simulink model "SF007A_SysFricLrng"  (R2013b)
settings: Solver=FixedStepDiscrete  SolverMode=SingleTasking  StartTime=0.0  StopTime=1  FixedStep=0.002  RelTol=1e-3
PostLoadFcn:
  | , if any(exist('dsrtsu_mdlpostloadfcn', 'file') == [2, 3, 6]), try dsrtsu_mdlpostloadfcn('Execute', bdroot); catch fprintf('Error in PostLoadFcn (dsrtsu_mdlpostloadfcn) for model "%s":\n %s\n', bdroot, lasterr); end, end,
undefined symbols (not defined in the file): ARCHGLBPRM_100MILLISEC_SEC_F32, ARCHGLBPRM_10MILLISEC_SEC_F32, ARCHGLBPRM_180OVERPI_ULS_F32, CONV100MICROSECTOSEC_ULS_F32, FLTINJ_SYSFRICLRNG_SYSFRICOFFS, FricLrngData, HiFricNtc, HWPTNUM_CNT_U08, HWPTNUMSUB1_CNT_U08, HWVELDECDIR_ULS_U08, HWVELINCDIR_ULS_U08, IDXCALCNSCAGFAC_ULS_U08, IDXSELN1_ULS_U08, IDXSELN2_ULS_U08, IDXSELN3_ULS_U08, LRNGENASCAFAC_MILLISEC_U32, NtcSts1, SCAGFACQUARTER_CNT_F32, SCAGFACTEN_CNT_U16, SECIDXSELN_ULS_U08, SysFricLrngBasLineEolFric, SysFricLrngBasLineFric, SysFricLrngBasLineHys, SysFricLrngBasLineRngCntr, SysFricLrngEolFricDifScagFac, SysFricLrngFricChgWght, SysFricLrngFricDiagcThd, SysFricLrngFricDiagcTiThd, SysFricLrngFricHysHwAgPt, SysFricLrngGain, SysFricLrngHwPosnAuthyThd, SysFricLrngHwVelConstrLim, SysFricLrngHwVelHiLim, SysFricLrngHwVelLoLim, SysFricLrngIgnCycFricChgLim, SysFricLrngLatAHiLim, SysFricLrngLatALoLim, SysFricLrngMaskVehSpd, SysFricLrngOperMod1, SysFricLrngRngCntrThd, SysFricLrngThd, SysFricLrngTHiLim, SysFricLrngTLoLim, SysFricLrngVehSpd, SYSFRICOFFSLIM_HWNWTMTR_F32, VEHSPDPTNUM1_ULS_U08, VEHSPDPTNUM2_ULS_U08
libraries: Fil x19, simulink x17, NxtrLim x10, NxtrAbslt x3, NxtrNvM x2, FixdToFloat x2, FloatToFixd x1, LnrIntrpn x1
(part 2 of 7)

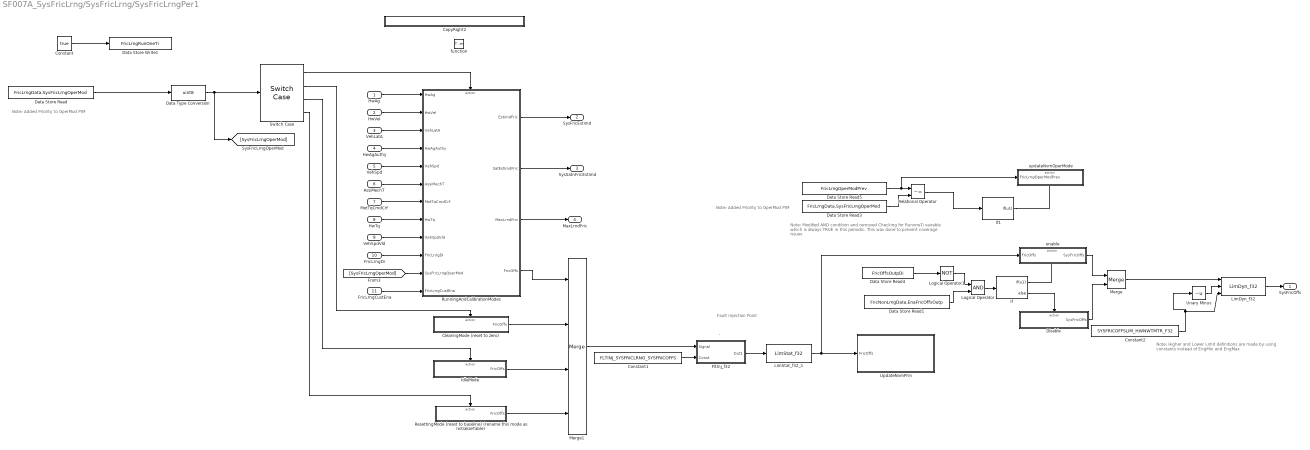
== system SF007A_SysFricLrng/SysFricLrng/SysFricLrngPer1 ==
  note: Note: Added Priority to OperMod PIM
  note: ,
  note: Fault
      | Injection
      | Point
  note: Note: Higher and Lower Limit definitions are made
      |           by using constants instead of EngMin and EngMax
  note: Note: Modified AND condition and removed Checking for RunoneTi
      | vairable which is always TRUE in this periodic. This was done to prevent
      | coverage issues
  note: Note: Added Priority to OperMod PIM
  HwAg : Inport
  HwVel : Inport  Port=2
  VehLatA : Inport  Port=3
  HwAgAuthy : Inport  Port=4
  VehSpd : Inport  Port=5
  AssiMechT : Inport  Port=6
  MotTqCmdCrf : Inport  Port=7
  HwTq : Inport  Port=8
  VehSpdVld : Inport  Port=9
  FricLrngDi : Inport  Port=10
  FricLrngCustEna : Inport  Port=11
  function : TriggerPort  TriggerType=function-call
  ClearingMode (reset to zero) : Subsystem
  Constant : Constant  Value=true  OutDataTypeStr=boolean
      settings: AttributesFormatString=%<OutDataTypeStr>
  Constant1 : Constant  Value=FLTINJ_SYSFRICLRNG_SYSFRICOFFS  SampleTime=-1
  Constant2 : Constant  Value=SYSFRICOFFSLIM_HWNWTMTR_F32  SampleTime=-1
  CopyRight2 : Subsystem  Description=|  mask(Copyright Information){none=on}
      | Copyright info block.                                               
      |                                                                     
      | Place copyright information at the top of every subsystem in design.
      mask prompts: none "No parameters"
      mask help: Place copyright information at the top of every subsystem in design.
      mask Display:
      | NxtrConf = 'Nexteer Confidential';
      | 
      | sys = bdroot; %handle for the current model ("system")
      | first = get_param(sys,'Created');
      | if(isempty(first))
      |     first = datestr(now,'yyyy');
      | else
      |     first = first(end-3:end);  %year is last four digits
      | end
      | 
      | last = get_param(sys,'LastModifiedDate');
      | if isempty(last)
      |     last = datestr(now,'yyyy');
      | else
      |     last = last(end-3:end);
      | end
      | 
      | if strcmp(first,last)
      |     fprintf('%s -- Copyright %s Nexteer',NxtrConf,first)
      | else
      |     fprintf('%s -- %s%s- %s Nexteer',NxtrConf,char(169),first,last)
      | end
  Data Store Read : DataStoreRead  Priority=1  DataStoreName=FricLrngData  DataStoreElements=FricLrngData.SysFricLrngOperMod
      settings: AttributesFormatString=Priority=%<Priority>
  Data Store Read1 : DataStoreRead  DataStoreName=FricNonLrngData  DataStoreElements=FricNonLrngData.EnaFricOffsOutp
  Data Store Read3 : DataStoreRead  Priority=2  DataStoreName=FricLrngData  DataStoreElements=FricLrngData.SysFricLrngOperMod
      settings: AttributesFormatString=Priority=%<Priority>
  Data Store Read4 : DataStoreRead  DataStoreName=FricOffsOutpDi
  Data Store Read5 : DataStoreRead  Priority=2  DataStoreName=FricLrngOperModPrev
  Data Store Write1 : DataStoreWrite  DataStoreName=FricLrngRunOneTi
  Data Type Conversion : DataTypeConversion  OutDataTypeStr=uint8
  Disable : Subsystem  TreatAsAtomicUnit=on
  FltInj_f32 : Subsystem  RequirementInfo={} %GIDa_0b9e84c1_4f47_4480_b4c5_5d0515f10b4a  TreatAsAtomicUnit=on  VariantControl=FltInj_sim  mask(Fault_Injection){}
      mask help: Fault Injection is a simulation only block for EA4 programs.
  IdleMode : Subsystem
  If : If  IfExpression=u1
  If1 : If  IfExpression=u1  ShowElse=off
  LimDyn_f32 : NxtrLim/LimDyn_f32
  LimStat_f32_1 : NxtrLim/LimStat_f32  LoLim=SysFricLrngFricOffsLoLim  HiLim=SysFricLrngFricOffsHiLim
      settings: AttributesFormatString=|
      | Low Limit: %<LoLim>
      | High Limit:%<HiLim>
  Logical Operator : Logic  AllPortsSameDT=off  OutDataTypeStr=boolean
  Logical Operator1 : Logic  Operator=NOT  AllPortsSameDT=off  OutDataTypeStr=boolean
  Merge : Merge
  Merge1 : Merge  Inputs=4
  Relational Operator : RelationalOperator  Operator=~=  OutDataTypeStr=boolean
  ResettingMode (reset to baseline) (rename this mode as InitializeTable) : Subsystem
  RunningAndCalibrationModes : Subsystem
  Switch Case : SwitchCase  CaseConditions={[0,1],2,3}
  Unary Minus : UnaryMinus
  UpdateNvmPrm : Subsystem
  enable : Subsystem  TreatAsAtomicUnit=on
  updateNvmOperMode : Subsystem  TreatAsAtomicUnit=on
  SysFricOffs : Outport
  SysFricEstimd : Outport  Port=2
  SysSatnFricEstimd : Outport  Port=3
  MaxLrndFric : Outport  Port=4
  wires:
  HwAg/1 -> RunningAndCalibrationModes/1(HwAg)
  HwVel/1 -> RunningAndCalibrationModes/2(HwVel)
  VehLatA/1 -> RunningAndCalibrationModes/3(VehLatA)
  HwAgAuthy/1 -> RunningAndCalibrationModes/4(HwAgAuthy)
  VehSpd/1 -> RunningAndCalibrationModes/5(VehSpd)
  AssiMechT/1 -> RunningAndCalibrationModes/6(AssiMechT)
  MotTqCmdCrf/1 -> RunningAndCalibrationModes/7(MotTqCmdCrf)
  HwTq/1 -> RunningAndCalibrationModes/8(HwTq)
  [SysFricLrngOperMod] -> RunningAndCalibrationModes/11(SysFricLrngOperMod)
  VehSpdVld/1 -> RunningAndCalibrationModes/9(VehSpdVld)
  Merge/1 -> LimDyn_f32/1
  Logical Operator1/1 -> Logical Operator/1
  Logical Operator/1 -> If/1
  LimStat_f32_1/1 -> enable/1(FricOffs), UpdateNvmPrm/1(FricOffs)
  Data Store Read1/1 -> Logical Operator/2
  FricLrngDi/1 -> RunningAndCalibrationModes/10(FricLrngDi)
  If/1 -> enable/Action
  If/2 -> Disable/Action
  enable/1("SysFricOffs ") -> Merge/1
  Disable/1(SysFricOffs) -> Merge/2
  Data Store Read/1 -> Data Type Conversion/1
  Switch Case/1 -> RunningAndCalibrationModes/Action
  Switch Case/2 -> ClearingMode (reset to zero)/Action
  Switch Case/3 -> IdleMode/Action
  Switch Case/4 -> ResettingMode (reset to baseline) (rename this mode as InitializeTable)/Action
  RunningAndCalibrationModes/4(FricOffs) -> Merge1/1
  ClearingMode (reset to zero)/1(FricOffs) -> Merge1/2
  IdleMode/1(FricOffs) -> Merge1/3
  ResettingMode (reset to baseline) (rename this mode as InitializeTable)/1(FricOffs) -> Merge1/4
  Data Type Conversion/1 -> Switch Case/1, [SysFricLrngOperMod]
  Merge1/1 -> FltInj_f32/1(Signal)
  FltInj_f32/1(Out1) -> LimStat_f32_1/1
  Constant1/1 -> FltInj_f32/2(Const)
  RunningAndCalibrationModes/2(SatEstimdFric) -> SysSatnFricEstimd/1
  RunningAndCalibrationModes/1(EstimdFric) -> SysFricEstimd/1
  FricLrngCustEna/1 -> RunningAndCalibrationModes/12(FricLrngCustEna)
  Data Store Read4/1 -> Logical Operator1/1
  Constant/1 -> Data Store Write1/1
  Data Store Read5/1 -> updateNvmOperMode/1(FricLrngOperModPrev), Relational Operator/1
  Data Store Read3/1 -> Relational Operator/2
  Relational Operator/1 -> If1/1
  If1/1 -> updateNvmOperMode/Action
  RunningAndCalibrationModes/3(MaxLrndFric) -> MaxLrndFric/1
  LimDyn_f32/1 -> SysFricOffs/1
  Unary Minus/1 -> LimDyn_f32/2
  Constant2/1 -> LimDyn_f32/3, Unary Minus/1

== system SF007A_SysFricLrng/call_SysFricLrngInit1/CopyRight2 ==

== system SF007A_SysFricLrng/call_SysFricLrngPer1/CopyRight2 ==

== system SF007A_SysFricLrng/SysFricLrng/ClrFricLrngOperMod/CopyRight2 ==

== system SF007A_SysFricLrng/SysFricLrng/GetFricData/CopyRight2 ==

== system SF007A_SysFricLrng/SysFricLrng/GetFricLrngData/CopyRight2 ==

== system SF007A_SysFricLrng/SysFricLrng/GetFricOffsOutpDi/CopyRight2 ==

== system SF007A_SysFricLrng/SysFricLrng/InitFricLrngTbl/CopyRight2 ==

== system SF007A_SysFricLrng/SysFricLrng/SetFricData/CopyRight2 ==

== system SF007A_SysFricLrng/SysFricLrng/SetFricLrngData/CopyRight2 ==

== system SF007A_SysFricLrng/SysFricLrng/SetFricOffsOutpDi/CopyRight2 ==

== system SF007A_SysFricLrng/SysFricLrng/SysFricLrngInit1/CopyRight2 ==

== system SF007A_SysFricLrng/SysFricLrng/SysFricLrngInit1/GetRefTmr100MicroSec32bit ==
  note: Created Aug 18, 2015
      | Modified Oct 21, 2015
      | Modified Oct 30, 2015
      | Kevin Derry
  note: GetRefTmr100MicroSec32bit
  note: Wrap-to-zero
  note: counts
  note: microseconds
  note: seconds
  note: 1 count = 100 uSec
  CopyRight2 : Subsystem  Description=|  mask(Copyright Information){none=on}
      | Copyright info block.                                               
      |                                                                     
      | Place copyright information at the top of every subsystem in design.
      mask prompts: none "No parameters"
      mask help: Place copyright information at the top of every subsystem in design.
      mask Display:
      | NxtrConf = 'Nexteer Confidential';
      | 
      | sys = bdroot; %handle for the current model ("system")
      | first = get_param(sys,'Created');
      | if(isempty(first))
      |     first = datestr(now,'yyyy');
      | else
      |     first = first(end-3:end);  %year is last four digits
      | end
      | 
      | last = get_param(sys,'LastModifiedDate');
      | if isempty(last)
      |     last = datestr(now,'yyyy');
      | else
      |     last = last(end-3:end);
      | end
      | 
      | if strcmp(first,last)
      |     fprintf('%s -- Copyright %s Nexteer',NxtrConf,first)
      | else
      |     fprintf('%s -- %s%s- %s Nexteer',NxtrConf,char(169),first,last)
      | end
  Count per uSec : Constant  Value=0.01
  Data Store Read1 : DataStoreRead  DataStoreName=SimnTi
  Data Type Conversion1 : DataTypeConversion  OutDataTypeStr=uint32
  Divide1 : Product  Inputs=**
  Divide2 : Product  Inputs=*/
  Max Counts : Constant  Value=2^32-1
  Product1 : Product
  Product2 : Product
  Rounding : Rounding
  Subtract1 : Sum  Inputs=+-
  uSec per Sec : Constant  Value=1000000
  RefTmr : Outport
  wires:
  Data Store Read1/1 -> Product1/1
  Data Type Conversion1/1 -> RefTmr/1
  uSec per Sec/1 -> Product1/2
  Count per uSec/1 -> Divide1/2
  Product1/1 -> Divide1/1
  Divide1/1 -> Subtract1/1, Divide2/1
  Max Counts/1 -> Product2/2, Divide2/2
  Divide2/1 -> Rounding/1
  Rounding/1 -> Product2/1
  Subtract1/1 -> Data Type Conversion1/1
  Product2/1 -> Subtract1/2

== system SF007A_SysFricLrng/SysFricLrng/SysFricLrngInit1/GetRefTmr100MicroSec32bit1 ==
  note: 1 count = 100 uSec
  note: seconds
  note: microseconds
  note: counts
  note: Wrap-to-zero
  note: GetRefTmr100MicroSec32bit
  note: Created Aug 18, 2015
      | Modified Oct 21, 2015
      | Modified Oct 30, 2015
      | Kevin Derry
  CopyRight2 : Subsystem  Description=|  mask(Copyright Information){none=on}
      | Copyright info block.                                               
      |                                                                     
      | Place copyright information at the top of every subsystem in design.
      mask prompts: none "No parameters"
      mask help: Place copyright information at the top of every subsystem in design.
      mask Display:
      | NxtrConf = 'Nexteer Confidential';
      | 
      | sys = bdroot; %handle for the current model ("system")
      | first = get_param(sys,'Created');
      | if(isempty(first))
      |     first = datestr(now,'yyyy');
      | else
      |     first = first(end-3:end);  %year is last four digits
      | end
      | 
      | last = get_param(sys,'LastModifiedDate');
      | if isempty(last)
      |     last = datestr(now,'yyyy');
      | else
      |     last = last(end-3:end);
      | end
      | 
      | if strcmp(first,last)
      |     fprintf('%s -- Copyright %s Nexteer',NxtrConf,first)
      | else
      |     fprintf('%s -- %s%s- %s Nexteer',NxtrConf,char(169),first,last)
      | end
  Count per uSec : Constant  Value=0.01
  Data Store Read1 : DataStoreRead  DataStoreName=SimnTi
  Data Type Conversion1 : DataTypeConversion  OutDataTypeStr=uint32
  Divide1 : Product  Inputs=**
  Divide2 : Product  Inputs=*/
  Max Counts : Constant  Value=2^32-1
  Product1 : Product
  Product2 : Product
  Rounding : Rounding
  Subtract1 : Sum  Inputs=+-
  uSec per Sec : Constant  Value=1000000
  RefTmr : Outport
  wires:
  Product2/1 -> Subtract1/2
  Subtract1/1 -> Data Type Conversion1/1
  Rounding/1 -> Product2/1
  Divide2/1 -> Rounding/1
  Max Counts/1 -> Divide2/2, Product2/2
  Divide1/1 -> Divide2/1, Subtract1/1
  Product1/1 -> Divide1/1
  Count per uSec/1 -> Divide1/2
  uSec per Sec/1 -> Product1/2
  Data Type Conversion1/1 -> RefTmr/1
  Data Store Read1/1 -> Product1/1

== system SF007A_SysFricLrng/SysFricLrng/SysFricLrngInit1/Initialization ==
  VEHSPDPTNUM1_ULS_U08 : Inport
  Assignment : Assignment  RequirementInfo={} %GIDa_e80d0eec_dc7b_46d2_bc23_1f2d78a3fae6  IndexOptions=Index vector (port)  Indices=1  OutputSizes=1
  Assignment1 : Assignment  RequirementInfo={} %GIDa_c9084e08_785a_4295_aaf7_90bdd84db3cf  IndexOptions=Index vector (port)  Indices=1  OutputSizes=1
  Assignment2 : Assignment  RequirementInfo={} %GIDa_524032d9_4688_4023_a955_e8523823905f  IndexOptions=Index vector (port)  Indices=1  OutputSizes=1
  Assignment3 : Assignment  RequirementInfo={} %GIDa_fab3be9c_982c_4710_b056_a8c629ce9d30  IndexOptions=Index vector (port)  Indices=1  OutputSizes=1
  Constant6 : Constant  Value=SysFricLrngBasLineFric
  CopyRight2 : Subsystem  Description=|  RequirementInfo={} %GIDa_9002c804_520f_46b6_95bc_d8cc45951013  mask(Copyright Information){none=on}
      | Copyright info block.                                               
      |                                                                     
      | Place copyright information at the top of every subsystem in design.
      mask prompts: none "No parameters"
      mask help: Place copyright information at the top of every subsystem in design.
      mask Display:
      | NxtrConf = 'Nexteer Confidential';
      | 
      | sys = bdroot; %handle for the current model ("system")
      | first = get_param(sys,'Created');
      | first = first(end-3:end);  %year is last four digits
      | 
      | last = get_param(sys,'LastModifiedDate');
      | if isempty(last)
      |     last = datestr(now,'yyyy');
      | else
      |     last = last(end-3:end);
      | end
      | 
      | if strcmp(first,last)
      |     fprintf('%s -- Copyright %s Nexteer',NxtrConf,first)
      | else
      |     fprintf('%s -- %s%s- %s Nexteer',NxtrConf,char(169),first,last)
      | end
  Data Store Read : DataStoreRead  DataStoreName=VehBasLineFric  DataStoreElements=VehBasLineFric
  Data Store Read1 : DataStoreRead  DataStoreName=RawAvrgFric  DataStoreElements=RawAvrgFric
  Data Store Read2 : DataStoreRead  DataStoreName=FilAvrgFric  DataStoreElements=FilAvrgFric
  Data Store Read3 : DataStoreRead  DataStoreName=SatnAvrgFric  DataStoreElements=SatnAvrgFric
  Data Store Read4 : DataStoreRead  DataStoreName=FricLrngData  DataStoreElements=FricLrngData.VehLrndFric(:,:)
  Data Store Write : DataStoreWrite  DataStoreName=VehBasLineFric
  Data Store Write3 : DataStoreWrite  DataStoreName=RawAvrgFric
  Data Store Write5 : DataStoreWrite  DataStoreName=FilAvrgFric
  Data Store Write7 : DataStoreWrite  DataStoreName=SatnAvrgFric
  For Iterator : ForIterator  RequirementInfo={} %GIDa_b61acb06_80c3_4c57_9830_a4b5c9b91ca4  IterationSource=external  IterationVariableDataType=int8
  InitAvrgFricLpFil1 : Subsystem
  InitAvrgFricLpFil2 : Subsystem
  InitAvrgFricLpFil3 : Subsystem
  InitAvrgFricLpFil4 : Subsystem
  Selector1 : Selector  InputPortWidth=4  IndexOptions=Index vector (port)  Indices=[1 3]  OutputSizes=1
  Selector2 : Selector  InputPortWidth=4  IndexOptions=Index vector (port)  Indices=[1 3]  OutputSizes=1
  Switch Case : SwitchCase  CaseConditions={1, 2, 3}
  wires:
  Constant6/1 -> Selector2/1
  For Iterator/1 -> [Idx], Selector2/2
  Selector2/1 -> Assignment/2
  Data Store Read/1 -> Assignment/1
  Data Store Read1/1 -> Assignment1/1
  Assignment1/1 -> Data Store Write3/1
  Data Store Read2/1 -> Assignment2/1
  Assignment2/1 -> Data Store Write5/1
  Data Store Read3/1 -> Assignment3/1
  Assignment3/1 -> Data Store Write7/1
  Selector1/1 -> InitAvrgFricLpFil1/1(VehLrndFric), InitAvrgFricLpFil2/1(VehLrndFric), InitAvrgFricLpFil4/1(VehLrndFric), InitAvrgFricLpFil3/1(VehLrndFric), Assignment3/2, Assignment2/2, Assignment1/2
  [Idx] -> Assignment/3
  [Idx] -> Assignment1/3
  [Idx] -> Assignment2/3
  [Idx] -> Assignment3/3
  [Idx] -> Selector1/2
  Data Store Read4/1 -> Selector1/1
  Assignment/1 -> Data Store Write/1
  VEHSPDPTNUM1_ULS_U08/1 -> For Iterator/1
  [Idx] -> Switch Case/1
  Switch Case/1 -> InitAvrgFricLpFil1/Action
  Switch Case/2 -> InitAvrgFricLpFil2/Action
  Switch Case/3 -> InitAvrgFricLpFil3/Action
  Switch Case/4 -> InitAvrgFricLpFil4/Action

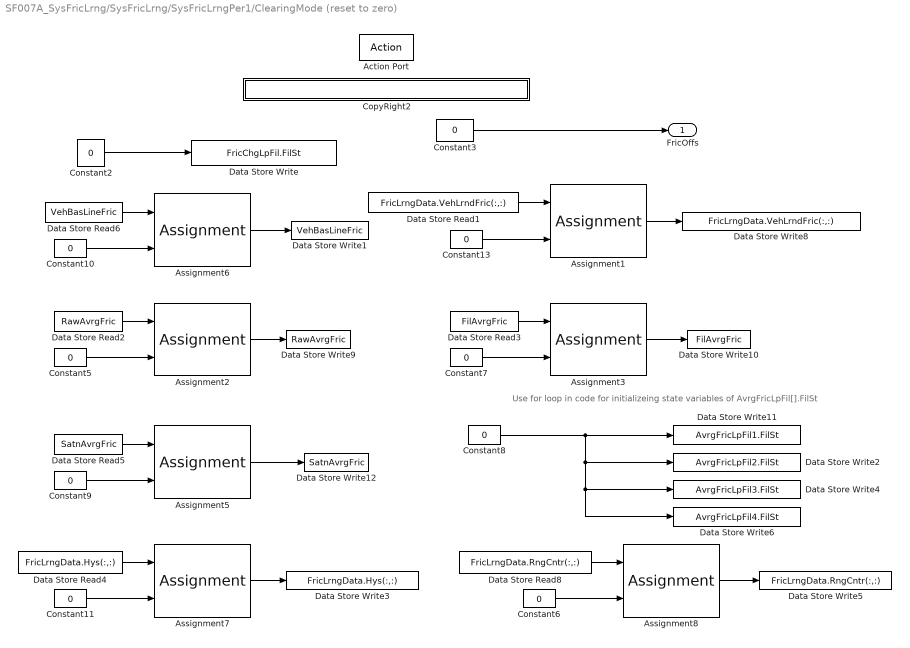
== system SF007A_SysFricLrng/SysFricLrng/SysFricLrngPer1/ClearingMode (reset to zero) ==
  note: Use for loop in code for initializeing state variables of AvrgFricLpFil[].FilSt
  Action Port : ActionPort  ActionType=case
  Assignment{1..3,5..6} (5 alike) : Assignment  IndexOptions=Assign all  Indices=1  OutputSizes=1
      settings: AttributesFormatString=Index: %<IndexOptions>
  Assignment7 : Assignment  NumberOfDimensions=2  IndexOptions=Assign all,Assign all  Indices=1,1  OutputSizes=1,1
      settings: AttributesFormatString=Index: %<IndexOptions>
  Assignment8 : Assignment  NumberOfDimensions=2  IndexOptions=Assign all,Assign all  Indices=1,1  OutputSizes=1,1
      settings: AttributesFormatString=Index: %<IndexOptions>
  Constant{2..3,5,7..11,13} (9 alike) : Constant  Value=0  OutDataTypeStr=single
      settings: AttributesFormatString=%<OutDataTypeStr>
  Constant6 : Constant  Value=0  OutDataTypeStr=uint16
      settings: AttributesFormatString=%<OutDataTypeStr>
  CopyRight2 : Subsystem  Description=|  mask(Copyright Information){none=on}
      | Copyright info block.                                               
      |                                                                     
      | Place copyright information at the top of every subsystem in design.
      mask prompts: none "No parameters"
      mask help: Place copyright information at the top of every subsystem in design.
      mask Display:
      | NxtrConf = 'Nexteer Confidential';
      | 
      | sys = bdroot; %handle for the current model ("system")
      | first = get_param(sys,'Created');
      | first = first(end-3:end);  %year is last four digits
      | 
      | last = get_param(sys,'LastModifiedDate');
      | if isempty(last)
      |     last = datestr(now,'yyyy');
      | else
      |     last = last(end-3:end);
      | end
      | 
      | if strcmp(first,last)
      |     fprintf('%s -- Copyright %s Nexteer',NxtrConf,first)
      | else
      |     fprintf('%s -- %s%s- %s Nexteer',NxtrConf,char(169),first,last)
      | end
  Data Store Read1 : DataStoreRead  Priority=1  DataStoreName=FricLrngData  DataStoreElements=FricLrngData.VehLrndFric(:,:)
      settings: AttributesFormatString=Priority: %<Priority>
  Data Store Read2 : DataStoreRead  Priority=1  DataStoreName=RawAvrgFric
      settings: AttributesFormatString=Priority: %<Priority>
  Data Store Read3 : DataStoreRead  Priority=1  DataStoreName=FilAvrgFric
      settings: AttributesFormatString=Priority: %<Priority>
  Data Store Read4 : DataStoreRead  Priority=1  DataStoreName=FricLrngData  DataStoreElements=FricLrngData.Hys(:,:)
      settings: AttributesFormatString=Priority: %<Priority>
  Data Store Read5 : DataStoreRead  Priority=1  DataStoreName=SatnAvrgFric
      settings: AttributesFormatString=Priority: %<Priority>
  Data Store Read6 : DataStoreRead  Priority=1  DataStoreName=VehBasLineFric
      settings: AttributesFormatString=Priority: %<Priority>
  Data Store Read8 : DataStoreRead  Priority=1  DataStoreName=FricLrngData  DataStoreElements=FricLrngData.RngCntr(:,:)
      settings: AttributesFormatString=Priority: %<Priority>
  Data Store Write : DataStoreWrite  DataStoreName=FricChgLpFil  DataStoreElements=FricChgLpFil.FilSt
  Data Store Write1 : DataStoreWrite  Priority=2  DataStoreName=VehBasLineFric
      settings: AttributesFormatString=Priority: %<Priority>
  Data Store Write10 : DataStoreWrite  Priority=2  DataStoreName=FilAvrgFric
      settings: AttributesFormatString=Priority: %<Priority>
  Data Store Write11 : DataStoreWrite  DataStoreName=AvrgFricLpFil1  DataStoreElements=AvrgFricLpFil1.FilSt
  Data Store Write12 : DataStoreWrite  Priority=2  DataStoreName=SatnAvrgFric
      settings: AttributesFormatString=Priority: %<Priority>
  Data Store Write2 : DataStoreWrite  DataStoreName=AvrgFricLpFil2  DataStoreElements=AvrgFricLpFil2.FilSt
  Data Store Write3 : DataStoreWrite  Priority=2  DataStoreName=FricLrngData  DataStoreElements=FricLrngData.Hys(:,:)
      settings: AttributesFormatString=Priority: %<Priority>
  Data Store Write4 : DataStoreWrite  DataStoreName=AvrgFricLpFil3  DataStoreElements=AvrgFricLpFil3.FilSt
  Data Store Write5 : DataStoreWrite  Priority=2  DataStoreName=FricLrngData  DataStoreElements=FricLrngData.RngCntr(:,:)
      settings: AttributesFormatString=Priority: %<Priority>
  Data Store Write6 : DataStoreWrite  DataStoreName=AvrgFricLpFil4  DataStoreElements=AvrgFricLpFil4.FilSt
  Data Store Write8 : DataStoreWrite  Priority=2  DataStoreName=FricLrngData  DataStoreElements=FricLrngData.VehLrndFric(:,:)
      settings: AttributesFormatString=Priority: %<Priority>
  Data Store Write9 : DataStoreWrite  Priority=2  DataStoreName=RawAvrgFric
      settings: AttributesFormatString=Priority: %<Priority>
  FricOffs : Outport  InitialOutput=[0]
  wires:
  Constant3/1 -> FricOffs/1
  Data Store Read1/1 -> Assignment1/1
  Constant13/1 -> Assignment1/2
  Assignment1/1 -> Data Store Write8/1
  Data Store Read2/1 -> Assignment2/1
  Constant5/1 -> Assignment2/2
  Assignment2/1 -> Data Store Write9/1
  Data Store Read3/1 -> Assignment3/1
  Constant7/1 -> Assignment3/2
  Assignment3/1 -> Data Store Write10/1
  Data Store Read5/1 -> Assignment5/1
  Constant9/1 -> Assignment5/2
  Assignment5/1 -> Data Store Write12/1
  Data Store Read6/1 -> Assignment6/1
  Constant10/1 -> Assignment6/2
  Assignment6/1 -> Data Store Write1/1
  Data Store Read4/1 -> Assignment7/1
  Assignment7/1 -> Data Store Write3/1
  Constant11/1 -> Assignment7/2
  Data Store Read8/1 -> Assignment8/1
  Assignment8/1 -> Data Store Write5/1
  Constant6/1 -> Assignment8/2
  Constant2/1 -> Data Store Write/1
  Constant8/1 -> Data Store Write2/1, Data Store Write4/1, Data Store Write6/1, Data Store Write11/1

== system SF007A_SysFricLrng/SysFricLrng/SysFricLrngPer1/CopyRight2 ==

== system SF007A_SysFricLrng/SysFricLrng/SysFricLrngPer1/Disable ==
  "Action Port " : ActionPort  ActionType=else
  Constant : Constant  Value=0  OutDataTypeStr=single
      settings: AttributesFormatString=%<OutDataTypeStr>
  CopyRight2 : Subsystem  Description=|  mask(Copyright Information){none=on}
      | Copyright info block.                                               
      |                                                                     
      | Place copyright information at the top of every subsystem in design.
      mask prompts: none "No parameters"
      mask help: Place copyright information at the top of every subsystem in design.
      mask Display:
      | NxtrConf = 'Nexteer Confidential';
      | 
      | sys = bdroot; %handle for the current model ("system")
      | first = get_param(sys,'Created');
      | first = first(end-3:end);  %year is last four digits
      | 
      | last = get_param(sys,'LastModifiedDate');
      | if isempty(last)
      |     last = datestr(now,'yyyy');
      | else
      |     last = last(end-3:end);
      | end
      | 
      | if strcmp(first,last)
      |     fprintf('%s -- Copyright %s Nexteer',NxtrConf,first)
      | else
      |     fprintf('%s -- %s%s- %s Nexteer',NxtrConf,char(169),first,last)
      | end
  SysFricOffs : Outport
  wires:
  Constant/1 -> SysFricOffs/1

== system SF007A_SysFricLrng/SysFricLrng/SysFricLrngPer1/FltInj_f32 ==
  note: Inport #2 must be constant
      | Const: FltInjectionLocType
  note: EA4.x Fault Injection
  note: This block requires no modification by FDD author.
      |
      | This block does not actually simulate any fault injection.  It is simply a pass-thru.
      |
      | The Const port (#2) simply terminates its signal, but we are trying to force the FDD author
      | to properly use the FltInjectionLocType enumeration in FDD model.
  Signal : Inport
  Const : Inport  Port=2
  Terminator : Terminator
  Out1 : Outport
  wires:
  Const/1 -> Terminator/1
  Signal/1 -> Out1/1

== system SF007A_SysFricLrng/SysFricLrng/SysFricLrngPer1/IdleMode ==
  note: Idle Mode means to do nothing new.
      |
      | Do not learn.
  Action Port : ActionPort  ActionType=case
  CopyRight2 : Subsystem  Description=|  mask(Copyright Information){none=on}
      | Copyright info block.                                               
      |                                                                     
      | Place copyright information at the top of every subsystem in design.
      mask prompts: none "No parameters"
      mask help: Place copyright information at the top of every subsystem in design.
      mask Display:
      | NxtrConf = 'Nexteer Confidential';
      | 
      | sys = bdroot; %handle for the current model ("system")
      | first = get_param(sys,'Created');
      | first = first(end-3:end);  %year is last four digits
      | 
      | last = get_param(sys,'LastModifiedDate');
      | if isempty(last)
      |     last = datestr(now,'yyyy');
      | else
      |     last = last(end-3:end);
      | end
      | 
      | if strcmp(first,last)
      |     fprintf('%s -- Copyright %s Nexteer',NxtrConf,first)
      | else
      |     fprintf('%s -- %s%s- %s Nexteer',NxtrConf,char(169),first,last)
      | end
  Data Store Read : DataStoreRead  DataStoreName=FricLrngData  DataStoreElements=FricLrngData.FricOffs
  FricOffs : Outport  InitialOutput=[0]
  wires:
  Data Store Read/1 -> FricOffs/1

== stateflow chart SF007A_SysFricLrng/SysFricLrng/SysFricLrngPer1/RunningAndCalibrationModes/FricLearning/Calculate Average Friction/NTC FAIL/NTCFAIL/SetNtcSts/SetNtcSts/ISO Fault Debounce Design ==
  note: NTCSTS_PASSD           (0)
      | NTCSTS_FAILD             (1)
      | NTCSTS_PREPASSD   (2)
      | NTCSTS_PREFAILD     (3)
      |
      | SIGQLFR_NORES        (0)
      | SIGQLFR_PASSD         (1)
      | SIGQLFR_FAILD           (2)
  note: Pass Loop
  note: Fail Loop
  note: 
  (default) -> (junction 89)
  (junction 89) -> (junction 95) [order 1] : [NtcSts ==3]
  (junction 89) -> (junction 93) [order 2] : [NtcSts ==2]
  (junction 89) -> (junction 141) [order 3] : [NtcSts ==1]
      | { ErrAcc = 32767;
      | Qualifier =2;
      |  }
  (junction 89) -> (junction 141) [order 4] : [NtcSts ==0]
      | { ErrAcc = -32768;
      | Qualifier=1;
      | }
  (junction 95) -> (junction 103) [order 2]
  (junction 95) -> (junction 111) [order 1] : [ErrAcc <=0]
      | {ErrAcc = DebStep;}
  (junction 93) -> (junction 123) [order 2] : {
      | ErrAcc = ErrAcc - DebStep;
      | }
  (junction 93) -> (junction 123) [order 1] : [(ErrAcc - DebStep) <= -32768]
      | { ErrAcc = -32768;
      | Qualifier=1;
      | }
  (junction 103) -> (junction 111) [order 1] : [(ErrAcc + DebStep) <32767]
      | {ErrAcc = ErrAcc + DebStep;}
  (junction 103) -> (junction 111) [order 2] : {ErrAcc = 32767;
      | Qualifier =2;}
  (junction 123) -> (junction 141)
  (junction 111) -> (junction 141)
  (junction 141) -> (junction 159) [order 2] : {ErrAcc = 0;
      | Qualifier =0;
      | }
  (junction 141) -> (junction 159) [order 1] : [SvcClr ==0]
  data: NtcSts input Enum: NtcSts1; Qualifier output uint8; DebStep input uint16; ErrAcc local single; SvcClr input

== system SF007A_SysFricLrng/SysFricLrng/SysFricLrngPer1/ResettingMode (reset to baseline) (rename this mode as InitializeTable) ==
  Action Port : ActionPort  ActionType=default
  Constant1 : Constant  Value=SysFricLrngBasLineEolFric
  Constant2 : Constant  Value=0  OutDataTypeStr=single
      settings: AttributesFormatString=%<OutDataTypeStr>
  Constant3 : Constant  Value=VEHSPDPTNUM1_ULS_U08
  Constant4 : Constant  Value=VEHSPDPTNUM2_ULS_U08
  Constant5 : Constant  Value=SysFricLrngEolFricDifScagFac
  CopyRight2 : Subsystem  Description=|  mask(Copyright Information){none=on}
      | Copyright info block.                                               
      |                                                                     
      | Place copyright information at the top of every subsystem in design.
      mask prompts: none "No parameters"
      mask help: Place copyright information at the top of every subsystem in design.
      mask Display:
      | NxtrConf = 'Nexteer Confidential';
      | 
      | sys = bdroot; %handle for the current model ("system")
      | first = get_param(sys,'Created');
      | first = first(end-3:end);  %year is last four digits
      | 
      | last = get_param(sys,'LastModifiedDate');
      | if isempty(last)
      |     last = datestr(now,'yyyy');
      | else
      |     last = last(end-3:end);
      | end
      | 
      | if strcmp(first,last)
      |     fprintf('%s -- Copyright %s Nexteer',NxtrConf,first)
      | else
      |     fprintf('%s -- %s%s- %s Nexteer',NxtrConf,char(169),first,last)
      | end
  Data Store Read2 : DataStoreRead  DataStoreName=FricNonLrngData  DataStoreElements=FricNonLrngData.EolFric
  Data Store Write : DataStoreWrite  DataStoreName=FricChgLpFil  DataStoreElements=FricChgLpFil.FilSt
  LimStat_f32 : NxtrLim/LimStat_f32  LoLim=SysFricLrngEolFricDifLoLim  HiLim=SysFricLrngEolFricDifHiLim
      settings: AttributesFormatString=|
      | Low Limit: %<LoLim>
      | High Limit:%<HiLim>
  Product : Product  RndMeth=Zero
  Sum : Sum  Inputs=+-
  UpdateBaselineFric : Subsystem  RequirementInfo={} %GIDa_5e175a40_2587_46e4_b1f6_fabef224c7ce  Priority=1  TreatAsAtomicUnit=on
  UpdateFricLrngHys_RngCntr : Subsystem  Priority=1  TreatAsAtomicUnit=on
  FricOffs : Outport  InitialOutput=[0]
  wires:
  Sum/1 -> Product/1
  Constant5/1 -> Product/2
  Product/1 -> LimStat_f32/1
  LimStat_f32/1 -> FricOffs/1, [EolFricDif]
  Data Store Read2/1 -> Sum/1
  Constant1/1 -> Sum/2
  [EolFricDif] -> UpdateBaselineFric/1(EolFricDif)
  [EolFricDif] -> UpdateFricLrngHys_RngCntr/1(EolFricDif)
  Constant2/1 -> Data Store Write/1
  Constant3/1 -> UpdateBaselineFric/2(VEHSPDPTNUM1_ULS_U08)
  Constant4/1 -> UpdateFricLrngHys_RngCntr/2(VEHSPDPTNUM2_ULS_U08)

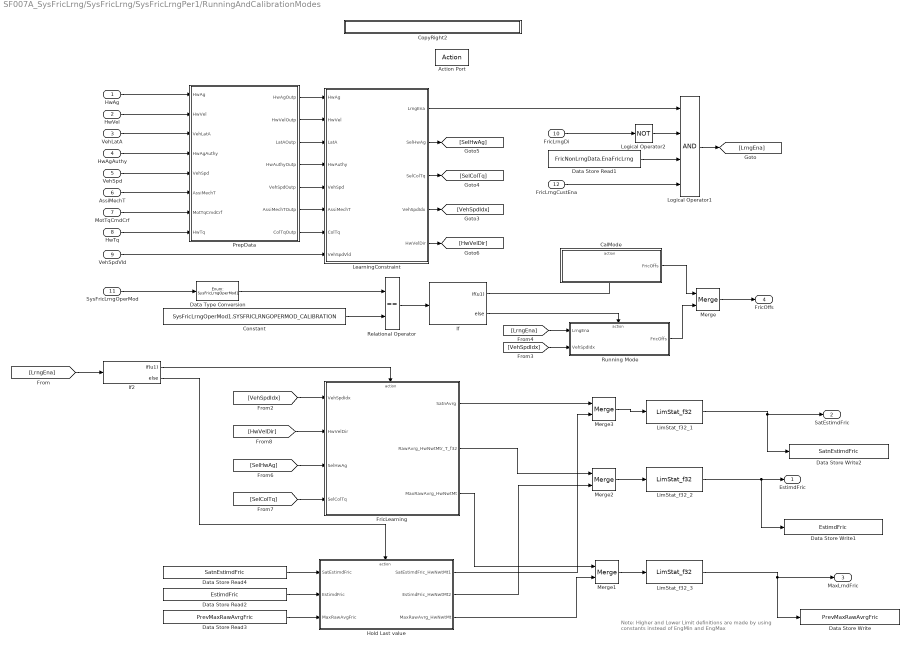
== system SF007A_SysFricLrng/SysFricLrng/SysFricLrngPer1/RunningAndCalibrationModes ==
  note: Note: Higher and Lower Limit definitions are made
      |           by using constants instead of EngMin and EngMax
  HwAg : Inport
  HwVel : Inport  Port=2
  VehLatA : Inport  Port=3
  HwAgAuthy : Inport  Port=4
  VehSpd : Inport  Port=5
  AssiMechT : Inport  Port=6
  MotTqCmdCrf : Inport  Port=7
  HwTq : Inport  Port=8
  VehSpdVld : Inport  Port=9
  FricLrngDi : Inport  Port=10
  SysFricLrngOperMod : Inport  Port=11
  FricLrngCustEna : Inport  Port=12
  Action Port : ActionPort  ActionType=case
  CalMode : Subsystem  TreatAsAtomicUnit=on
  Constant : Constant  Value=SysFricLrngOperMod1.SYSFRICLRNGOPERMOD_CALIBRATION  OutDataTypeStr=Enum: SysFricLrngOperMod1
      settings: AttributesFormatString=%<OutDataTypeStr>
  CopyRight2 : Subsystem  Description=|  mask(Copyright Information){none=on}
      | Copyright info block.                                               
      |                                                                     
      | Place copyright information at the top of every subsystem in design.
      mask prompts: none "No parameters"
      mask help: Place copyright information at the top of every subsystem in design.
      mask Display:
      | NxtrConf = 'Nexteer Confidential';
      | 
      | sys = bdroot; %handle for the current model ("system")
      | first = get_param(sys,'Created');
      | first = first(end-3:end);  %year is last four digits
      | 
      | last = get_param(sys,'LastModifiedDate');
      | if isempty(last)
      |     last = datestr(now,'yyyy');
      | else
      |     last = last(end-3:end);
      | end
      | 
      | if strcmp(first,last)
      |     fprintf('%s -- Copyright %s Nexteer',NxtrConf,first)
      | else
      |     fprintf('%s -- %s%s- %s Nexteer',NxtrConf,char(169),first,last)
      | end
  Data Store Read1 : DataStoreRead  DataStoreName=FricNonLrngData  DataStoreElements=FricNonLrngData.EnaFricLrng
  Data Store Read2 : DataStoreRead  Priority=1  DataStoreName=EstimdFric
      settings: AttributesFormatString=Priority: %<Priority>
  Data Store Read3 : DataStoreRead  Priority=1  DataStoreName=PrevMaxRawAvrgFric
      settings: AttributesFormatString=Priority: %<Priority>
  Data Store Read4 : DataStoreRead  Priority=1  DataStoreName=SatnEstimdFric
      settings: AttributesFormatString=Priority: %<Priority>
  Data Store Write : DataStoreWrite  Priority=2  DataStoreName=PrevMaxRawAvrgFric
      settings: AttributesFormatString=Priority:%<Priority>
  Data Store Write1 : DataStoreWrite  Priority=2  DataStoreName=EstimdFric
      settings: AttributesFormatString=Priority:%<Priority>
  Data Store Write2 : DataStoreWrite  Priority=2  DataStoreName=SatnEstimdFric
      settings: AttributesFormatString=Priority:%<Priority>
  Data Type Conversion : DataTypeConversion  OutDataTypeStr=Enum: SysFricLrngOperMod1
  FricLearning : Subsystem
  Hold Last value : Subsystem
  If : If  IfExpression=u1
  If2 : If  IfExpression=u1
  LearningConstraint : Subsystem
  LimStat_f32_1 : NxtrLim/LimStat_f32  LoLim=SYSSATNFRICESTIMDLOLIM_HWNWTMTR_F32  HiLim=SYSSATNFRICESTIMDHILIM_HWNWTMTR_F32
      settings: AttributesFormatString=|
      | Low Limit: %<LoLim>
      | High Limit:%<HiLim>
  LimStat_f32_2 : NxtrLim/LimStat_f32  LoLim=SYSFRICESTIMDLOLIM_HWNWTMTR_F32  HiLim=SYSFRICESTIMDHILIM_HWNWTMTR_F32
      settings: AttributesFormatString=|
      | Low Limit: %<LoLim>
      | High Limit:%<HiLim>
  LimStat_f32_3 : NxtrLim/LimStat_f32  LoLim=MAXLRNDFRICLOLIM_HWNWTMTR_F32  HiLim=MAXLRNDFRICHILIM_HWNWTMTR_F32
      settings: AttributesFormatString=|
      | Low Limit: %<LoLim>
      | High Limit:%<HiLim>
  Logical Operator1 : Logic  Inputs=4  AllPortsSameDT=off  OutDataTypeStr=boolean
  Logical Operator2 : Logic  Operator=NOT  AllPortsSameDT=off  OutDataTypeStr=boolean
  Merge{,1..3} (4 alike) : Merge
  PrepData : Subsystem
  Relational Operator : RelationalOperator  Operator===  OutDataTypeStr=boolean
  Running Mode : Subsystem  TreatAsAtomicUnit=on
  EstimdFric : Outport
  SatEstimdFric : Outport  Port=2
  MaxLrndFric : Outport  Port=3
  FricOffs : Outport  Port=4
  wires:
  LearningConstraint/4(VehSpdIdx) -> [VehSpdIdx]
  LearningConstraint/3(SelColTq) -> [SelColTq]
  LearningConstraint/2(SelHwAg) -> [SelHwAg]
  PrepData/1(HwAgOutp) -> LearningConstraint/1(HwAg)
  PrepData/2(HwVelOutp) -> LearningConstraint/2(HwVel)
  HwAg/1 -> PrepData/1(HwAg)
  HwVel/1 -> PrepData/2(HwVel)
  VehLatA/1 -> PrepData/3(VehLatA)
  HwAgAuthy/1 -> PrepData/4(HwAgAuthy)
  VehSpd/1 -> PrepData/5(VehSpd)
  AssiMechT/1 -> PrepData/6(AssiMechT)
  MotTqCmdCrf/1 -> PrepData/7(MotTqCmdCrf)
  HwTq/1 -> PrepData/8(HwTq)
  LearningConstraint/5(HwVelDir) -> [HwVelDir]
  PrepData/3(LatAOutp) -> LearningConstraint/3(LatA)
  PrepData/4(HwAuthyOutp) -> LearningConstraint/4(HwAuthy)
  PrepData/5(VehSpdOutp) -> LearningConstraint/5(VehSpd)
  PrepData/6(AssiMechTOutp) -> LearningConstraint/6(AssiMechT)
  PrepData/7(ColTqOutp) -> LearningConstraint/7(ColTq)
  VehSpdVld/1 -> LearningConstraint/8(VehSpdVld)
  FricLrngDi/1 -> Logical Operator2/1
  LearningConstraint/1(LrngEna) -> Logical Operator1/1
  Merge/1 -> FricOffs/1
  [LrngEna] -> If2/1
  FricLrngCustEna/1 -> Logical Operator1/4
  [VehSpdIdx] -> FricLearning/1(VehSpdIdx)
  [HwVelDir] -> FricLearning/2(HwVelDir)
  [SelHwAg] -> FricLearning/3(SelHwAg)
  [SelColTq] -> FricLearning/4(SelColTq)
  SysFricLrngOperMod/1 -> Data Type Conversion/1
  Constant/1 -> Relational Operator/2
  Relational Operator/1 -> If/1
  Logical Operator1/1 -> [LrngEna]
  If/1 -> CalMode/Action
  CalMode/1(FricOffs) -> Merge/1
  Running Mode/1(FricOffs) -> Merge/2
  Data Type Conversion/1 -> Relational Operator/1
  Logical Operator2/1 -> Logical Operator1/2
  Data Store Read1/1 -> Logical Operator1/3
  If/2 -> Running Mode/Action
  [VehSpdIdx] -> Running Mode/2(VehSpdIdx)
  [LrngEna] -> Running Mode/1(LrngEna)
  Hold Last value/3(MaxRawAvrg_HwNwtMt) -> Merge1/2
  If2/1 -> FricLearning/Action
  Merge1/1 -> LimStat_f32_3/1
  FricLearning/3(MaxRawAvrg_HwNwtMt) -> Merge1/1
  If2/2 -> Hold Last value/Action
  Data Store Read3/1 -> Hold Last value/3(MaxRawAvgFric)
  Data Store Read4/1 -> Hold Last value/1(SatEstimdFric)
  Data Store Read2/1 -> Hold Last value/2(EstimdFric)
  LimStat_f32_1/1 -> Data Store Write2/1, SatEstimdFric/1
  FricLearning/1(SatnAvrg) -> Merge3/1
  Hold Last value/1(SatEstimdFric_HwNwtMt1) -> Merge3/2
  Hold Last value/2(EstimdFric_HwNwtMt2) -> Merge2/2
  FricLearning/2(RawAvrg_HwNwtMtr_T_f32) -> Merge2/1
  LimStat_f32_2/1 -> Data Store Write1/1, EstimdFric/1
  Merge3/1 -> LimStat_f32_1/1
  Merge2/1 -> LimStat_f32_2/1
  LimStat_f32_3/1 -> Data Store Write/1, MaxLrndFric/1

== system SF007A_SysFricLrng/SysFricLrng/SysFricLrngPer1/UpdateNvmPrm ==
  note: Set Ram Block Status for 'FricLrngData' moved to Init
  FricOffs : Inport
  Constant1 : Constant  Value=VEHSPDPTNUM1_ULS_U08
  CopyRight2 : Subsystem  Description=|  mask(Copyright Information){none=on}
      | Copyright info block.                                               
      |                                                                     
      | Place copyright information at the top of every subsystem in design.
      mask prompts: none "No parameters"
      mask help: Place copyright information at the top of every subsystem in design.
      mask Display:
      | NxtrConf = 'Nexteer Confidential';
      | 
      | sys = bdroot; %handle for the current model ("system")
      | first = get_param(sys,'Created');
      | if(isempty(first))
      |     first = datestr(now,'yyyy');
      | else
      |     first = first(end-3:end);  %year is last four digits
      | end
      | 
      | last = get_param(sys,'LastModifiedDate');
      | if isempty(last)
      |     last = datestr(now,'yyyy');
      | else
      |     last = last(end-3:end);
      | end
      | 
      | if strcmp(first,last)
      |     fprintf('%s -- Copyright %s Nexteer',NxtrConf,first)
      | else
      |     fprintf('%s -- %s%s- %s Nexteer',NxtrConf,char(169),first,last)
      | end
  Data Store Write1 : DataStoreWrite  DataStoreName=FricLrngData  DataStoreElements=FricLrngData.FricOffs
  UpdateVehLearnedFric : Subsystem  TreatAsAtomicUnit=on
  wires:
  FricOffs/1 -> Data Store Write1/1
  Constant1/1 -> UpdateVehLearnedFric/1(ItrnLim)

== system SF007A_SysFricLrng/SysFricLrng/SysFricLrngPer1/enable ==
  FricOffs : Inport
  Action Port : ActionPort  ActionType=then
  CopyRight2 : Subsystem  Description=|  mask(Copyright Information){none=on}
      | Copyright info block.                                               
      |                                                                     
      | Place copyright information at the top of every subsystem in design.
      mask prompts: none "No parameters"
      mask help: Place copyright information at the top of every subsystem in design.
      mask Display:
      | NxtrConf = 'Nexteer Confidential';
      | 
      | sys = bdroot; %handle for the current model ("system")
      | first = get_param(sys,'Created');
      | first = first(end-3:end);  %year is last four digits
      | 
      | last = get_param(sys,'LastModifiedDate');
      | if isempty(last)
      |     last = datestr(now,'yyyy');
      | else
      |     last = last(end-3:end);
      | end
      | 
      | if strcmp(first,last)
      |     fprintf('%s -- Copyright %s Nexteer',NxtrConf,first)
      | else
      |     fprintf('%s -- %s%s- %s Nexteer',NxtrConf,char(169),first,last)
      | end
  "SysFricOffs " : Outport
  wires:
  FricOffs/1 -> "SysFricOffs "/1

== system SF007A_SysFricLrng/SysFricLrng/SysFricLrngPer1/updateNvmOperMode ==
  note: Set Ram Block Status for 'FricLrngData' moved to Init
  FricLrngOperModPrev : Inport
  Action Port : ActionPort  ActionType=then
  CopyRight2 : Subsystem  Description=|  mask(Copyright Information){none=on}
      | Copyright info block.                                               
      |                                                                     
      | Place copyright information at the top of every subsystem in design.
      mask prompts: none "No parameters"
      mask help: Place copyright information at the top of every subsystem in design.
      mask Display:
      | NxtrConf = 'Nexteer Confidential';
      | 
      | sys = bdroot; %handle for the current model ("system")
      | first = get_param(sys,'Created');
      | first = first(end-3:end);  %year is last four digits
      | 
      | last = get_param(sys,'LastModifiedDate');
      | if isempty(last)
      |     last = datestr(now,'yyyy');
      | else
      |     last = last(end-3:end);
      | end
      | 
      | if strcmp(first,last)
      |     fprintf('%s -- Copyright %s Nexteer',NxtrConf,first)
      | else
      |     fprintf('%s -- %s%s- %s Nexteer',NxtrConf,char(169),first,last)
      | end
  Data Store Write1 : DataStoreWrite  DataStoreName=FricLrngData  DataStoreElements=FricLrngData.SysFricLrngOperMod
  wires:
  FricLrngOperModPrev/1 -> Data Store Write1/1

== system SF007A_SysFricLrng/SysFricLrng/SysFricLrngInit1/GetRefTmr100MicroSec32bit/CopyRight2 ==

== system SF007A_SysFricLrng/SysFricLrng/SysFricLrngInit1/GetRefTmr100MicroSec32bit1/CopyRight2 ==

== system SF007A_SysFricLrng/SysFricLrng/SysFricLrngInit1/Initialization/CopyRight2 ==

== system SF007A_SysFricLrng/SysFricLrng/SysFricLrngInit1/Initialization/InitAvrgFricLpFil1 ==
  VehLrndFric : Inport
  Action Port : ActionPort  ActionType=case
  CopyRight2 : Subsystem  Description=|  mask(Copyright Information){none=on}
      | Copyright info block.                                               
      |                                                                     
      | Place copyright information at the top of every subsystem in design.
      mask prompts: none "No parameters"
      mask help: Place copyright information at the top of every subsystem in design.
      mask Display:
      | NxtrConf = 'Nexteer Confidential';
      | 
      | sys = bdroot; %handle for the current model ("system")
      | first = get_param(sys,'Created');
      | first = first(end-3:end);  %year is last four digits
      | 
      | last = get_param(sys,'LastModifiedDate');
      | if isempty(last)
      |     last = datestr(now,'yyyy');
      | else
      |     last = last(end-3:end);
      | end
      | 
      | if strcmp(first,last)
      |     fprintf('%s -- Copyright %s Nexteer',NxtrConf,first)
      | else
      |     fprintf('%s -- %s%s- %s Nexteer',NxtrConf,char(169),first,last)
      | end
  Data Store Write : DataStoreWrite  DataStoreName=AvrgFricLpFil1  DataStoreElements=AvrgFricLpFil1.FilSt
  wires:
  VehLrndFric/1 -> Data Store Write/1

== system SF007A_SysFricLrng/SysFricLrng/SysFricLrngInit1/Initialization/InitAvrgFricLpFil2 ==
  VehLrndFric : Inport
  Action Port : ActionPort  ActionType=case
  CopyRight2 : Subsystem  Description=|  mask(Copyright Information){none=on}
      | Copyright info block.                                               
      |                                                                     
      | Place copyright information at the top of every subsystem in design.
      mask prompts: none "No parameters"
      mask help: Place copyright information at the top of every subsystem in design.
      mask Display:
      | NxtrConf = 'Nexteer Confidential';
      | 
      | sys = bdroot; %handle for the current model ("system")
      | first = get_param(sys,'Created');
      | first = first(end-3:end);  %year is last four digits
      | 
      | last = get_param(sys,'LastModifiedDate');
      | if isempty(last)
      |     last = datestr(now,'yyyy');
      | else
      |     last = last(end-3:end);
      | end
      | 
      | if strcmp(first,last)
      |     fprintf('%s -- Copyright %s Nexteer',NxtrConf,first)
      | else
      |     fprintf('%s -- %s%s- %s Nexteer',NxtrConf,char(169),first,last)
      | end
  Data Store Write : DataStoreWrite  DataStoreName=AvrgFricLpFil2  DataStoreElements=AvrgFricLpFil2.FilSt
  wires:
  VehLrndFric/1 -> Data Store Write/1

== system SF007A_SysFricLrng/SysFricLrng/SysFricLrngInit1/Initialization/InitAvrgFricLpFil3 ==
  VehLrndFric : Inport
  Action Port : ActionPort  ActionType=case
  CopyRight2 : Subsystem  Description=|  mask(Copyright Information){none=on}
      | Copyright info block.                                               
      |                                                                     
      | Place copyright information at the top of every subsystem in design.
      mask prompts: none "No parameters"
      mask help: Place copyright information at the top of every subsystem in design.
      mask Display:
      | NxtrConf = 'Nexteer Confidential';
      | 
      | sys = bdroot; %handle for the current model ("system")
      | first = get_param(sys,'Created');
      | first = first(end-3:end);  %year is last four digits
      | 
      | last = get_param(sys,'LastModifiedDate');
      | if isempty(last)
      |     last = datestr(now,'yyyy');
      | else
      |     last = last(end-3:end);
      | end
      | 
      | if strcmp(first,last)
      |     fprintf('%s -- Copyright %s Nexteer',NxtrConf,first)
      | else
      |     fprintf('%s -- %s%s- %s Nexteer',NxtrConf,char(169),first,last)
      | end
  Data Store Write : DataStoreWrite  DataStoreName=AvrgFricLpFil3  DataStoreElements=AvrgFricLpFil3.FilSt
  wires:
  VehLrndFric/1 -> Data Store Write/1

== system SF007A_SysFricLrng/SysFricLrng/SysFricLrngInit1/Initialization/InitAvrgFricLpFil4 ==
  VehLrndFric : Inport
  Action Port : ActionPort  ActionType=default
  CopyRight2 : Subsystem  Description=|  mask(Copyright Information){none=on}
      | Copyright info block.                                               
      |                                                                     
      | Place copyright information at the top of every subsystem in design.
      mask prompts: none "No parameters"
      mask help: Place copyright information at the top of every subsystem in design.
      mask Display:
      | NxtrConf = 'Nexteer Confidential';
      | 
      | sys = bdroot; %handle for the current model ("system")
      | first = get_param(sys,'Created');
      | first = first(end-3:end);  %year is last four digits
      | 
      | last = get_param(sys,'LastModifiedDate');
      | if isempty(last)
      |     last = datestr(now,'yyyy');
      | else
      |     last = last(end-3:end);
      | end
      | 
      | if strcmp(first,last)
      |     fprintf('%s -- Copyright %s Nexteer',NxtrConf,first)
      | else
      |     fprintf('%s -- %s%s- %s Nexteer',NxtrConf,char(169),first,last)
      | end
  Data Store Write : DataStoreWrite  DataStoreName=AvrgFricLpFil4  DataStoreElements=AvrgFricLpFil4.FilSt
  wires:
  VehLrndFric/1 -> Data Store Write/1

== system SF007A_SysFricLrng/SysFricLrng/SysFricLrngPer1/ClearingMode (reset to zero)/CopyRight2 ==

== system SF007A_SysFricLrng/SysFricLrng/SysFricLrngPer1/Disable/CopyRight2 ==

== system SF007A_SysFricLrng/SysFricLrng/SysFricLrngPer1/IdleMode/CopyRight2 ==

== system SF007A_SysFricLrng/SysFricLrng/SysFricLrngPer1/ResettingMode (reset to baseline) (rename this mode as InitializeTable)/CopyRight2 ==
